simulink model "project1"  (R2020b)
settings: Solver=VariableStepAuto  StartTime=0.0  StopTime=10.0  RelTol=1e-3
settings Model: Creator=k.Raviteja  LastModifiedBy=k.Raviteja

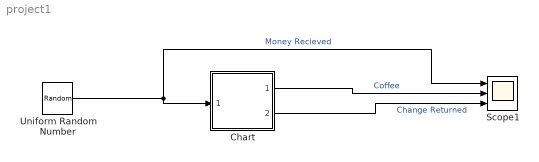
== system project1 ==
  Chart : Stateflow chart  TreatAsAtomicUnit=on
  Scope1 : Scope  NumInputPorts=3
  Uniform Random Number : UniformRandomNumber  Minimum=0  Maximum=20  SampleTime=0.5
  wires:
  Chart/1(Coffee) -> Scope1/2  "Coffee"
  Uniform Random Number/1 -> Scope1/1, Chart/1(money)  "Money Recieved"
  Chart/2(change) -> Scope1/3  "Change Returned"

== stateflow chart project1/Chart ==
  state checking_for_money
  state Got_money
  (default) -> checking_for_money
  checking_for_money -> Got_money : [money>=10]{Coffee=1;change=money-10;}
  Got_money -> checking_for_money : [money<10]{Coffee=0;}
  data: Coffee output double; money input; change output
